simulink model "quadFly"  (R2019b)
settings: Solver=ode4  StartTime=0.0  StopTime=inf  FixedStep=0.001  RelTol=1e-3
InitFcn:
  | Init_control;
values from neighbouring files (symbols this model uses):
  Kd_RP_AgngleRate = 0.005    [Init_control.m]    (also in quadFly.sldd)
  Kd_YAW_AngleRate = 0.05    [Init_control.m]    (also in quadFly.sldd)
  Ki_RP_AgngleRate = 0.01    [Init_control.m]    (also in quadFly.sldd)
  Ki_YAW_AngleRate = 0.8    [Init_control.m]    (also in quadFly.sldd)
  Kp_RP_AgngleRate = 0.55    [Init_control.m]    (also in quadFly.sldd)
  Kp_RP_ANGLE = 6.5    [Init_control.m]    (also in quadFly.sldd)
  Kp_YAW_AngleRate = 3.2    [Init_control.m]    (also in quadFly.sldd)
  MAX_CONTROL_ANGLE_RATE_Y = 90    [Init_control.m]    (also in quadFly.sldd = 90.0)
  ModelInit_RPM = 0.0    [quadFly.sldd]
  ModelParam_envAltitude = -41.5260009765625    [quadFly.sldd]
  ModelParam_GlobalNoiseGainSwitch = 1.0    [quadFly.sldd]
  ModelParam_GPSLatLong = 40.1540302 116.2593683    [quadFly.sldd]
  ModelParam_motorCr = 1148.0    [quadFly.sldd]
  ModelParam_motorJm = 0.0001287    [quadFly.sldd]
  ModelParam_motorMinThr = 0.05    [quadFly.sldd]
  ModelParam_motorT = 0.02    [quadFly.sldd]
  ModelParam_motorWb = -141.4    [quadFly.sldd]
  ModelParam_rotorCm = 1.779E-7    [quadFly.sldd]
  ModelParam_rotorCt = 1.105E-5    [quadFly.sldd]
  ModelParam_uavCCm = 0.01 0.01 0.0055    [quadFly.sldd]
  ModelParam_uavCd = 0.073    [quadFly.sldd]
  ModelParam_uavDearo = 0.12    [quadFly.sldd]
  ModelParam_uavJ = 0.0211 0.0 0.0 0.0 0.0219 0.0 0.0 0.0 0.0366    [quadFly.sldd]
  ModelParam_uavMass = 1.4    [quadFly.sldd]
  ModelParam_uavR = 0.225    [quadFly.sldd]
  ModelParam_uavType = 3    [quadFly.sldd]
undefined symbols (not defined in the file or in its folder): DWORK0, DWORK1, DWORK10, DWORK11, DWORK12, DWORK13, DWORK14, DWORK15, DWORK2, DWORK3, DWORK4, DWORK5, DWORK6, DWORK7, DWORK8, DWORK9, earthRadius, KiPitchAttitude, KiRollAttitude, Receive, Send
libraries: simulink x15, ctrl_ADRC_angular_rate x4, aerolibfltsims x3, ctrl_ADRC_TD x2, shared6dof x1, aerolibanimutils x1
(part 1 of 4)
settings Model: DataDictionary=quadFly.sldd  SimulationMode=accelerator  Creator=dream  LastModifiedBy=75696
settings DataIOCC: ReturnWorkspaceOutputs=off
settings DebuggingCC: BusObjectLabelMismatch=error  ArithmeticOperatorsInVariantConditions=warning
settings SFSimCC: SimUseLocalCustomCode=off  CustomCodeUndefinedFunction=UseInterfaceOnly
settings RTWCC: RTWUseLocalCustomCode=off
settings CodeAppCC: StateflowObjectComments=on

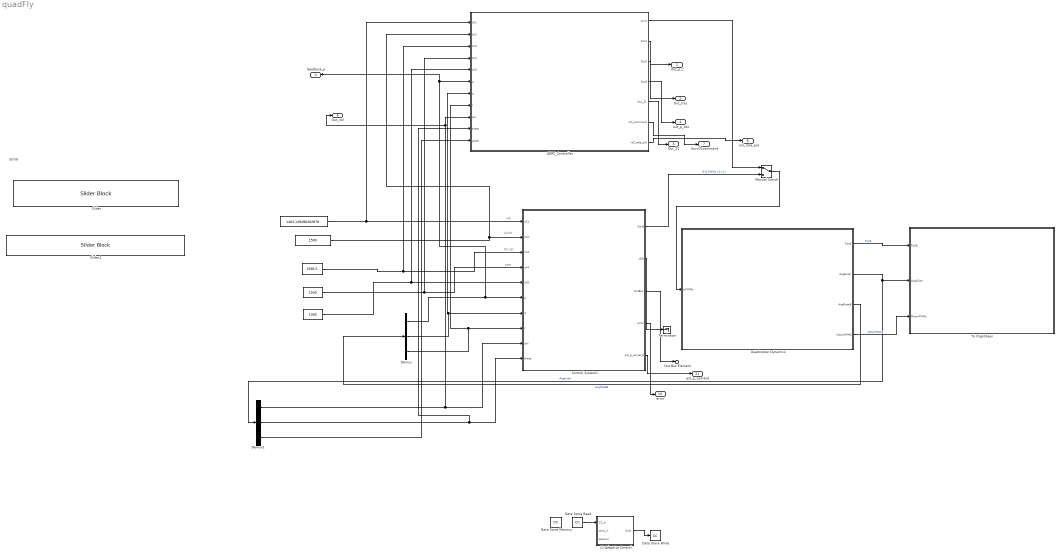
== system quadFly ==
  note: 遥控器
  note: roll
  note: pitch
  note: thrust
  note: yaw
  " " : Constant  Value=1000  OutDataTypeStr=uint16
  "  " : Constant  Value=1500  OutDataTypeStr=uint16
  "   " : Constant  Value=1463.129496402878  OutDataTypeStr=uint16
  "      " : Constant  Value=1596.5  OutDataTypeStr=uint16
  "          " : Constant  Value=1500  OutDataTypeStr=uint16
  "ADRC_Controller " : Subsystem
      mask Display: image('v2-31b439c605ff7f3f51fcae1000b27190_1440w.jpg'); % Use "Edit Image" on toolstrip to change.
  Control System1 : Subsystem
      mask Display: image('icon\pixhawk.png');
  Data Store Memory : DataStoreMemory  DataStoreName=CC  ReadBeforeWriteMsg=warning  WriteAfterWriteMsg=warning  WriteAfterReadMsg=warning  InitialValue=c2init  ShowAdditionalParam=off
  Data Store Read : DataStoreRead  DataStoreName=CC
  Data Store Write : DataStoreWrite  DataStoreName=CC
  Demux : Demux  Outputs=3
  Demux1 : Demux  Outputs=3
  L1-Adaptive Control : Subsystem
  Manual Switch : ManualSwitch
  Quadcopter Dynamics : Subsystem
      mask Display: image('icon/F450.png');
  Slider : SliderBlock  ScaleMin=1100  ScaleMax=1900
  Slider2 : SliderBlock  ScaleMin=1100  ScaleMax=1900
  Terminator : Terminator
  To FlightGear : Subsystem
      mask Display: image('icon/FlightGear.png');
  Out_p_c : Outport
  Out_trac : Outport  Port=2
  feedback_p : Outport  Port=3
  out_p_dot : Outport  Port=4
  Out_Z1 : Outport  Port=5
  Out_roll : Outport  Port=6
  Ouroll1command : Outport  Port=7
  roll_rate_pid : Outport  Port=8
  Out Bus Element : Outport  Port=9  PortName=OutBus  Element=signal1
  error : Outport  Port=10
  pid_p_comand : Outport  Port=11
  wires:
  Quadcopter Dynamics/1(PosE) -> To FlightGear/1(PosE)  "PosE"
  Control System1/2(LED) -> Terminator/1
  Quadcopter Dynamics/2(AngEuler) -> To FlightGear/2(AngEular), Demux1/1  "AngEular"
  "   "/1 -> Control System1/1(ch1), "ADRC_Controller "/1(ch1)
  "          "/1 -> Control System1/4(ch4), "ADRC_Controller "/4(ch4)
  "      "/1 -> "ADRC_Controller "/3(ch3), Control System1/3(ch3)
  Quadcopter Dynamics/3(AngRateB) -> Demux/1  "AngRateB"
  " "/1 -> "ADRC_Controller "/5(ch5), Control System1/5(ch5)
  Demux/1 -> feedback_p/1, "ADRC_Controller "/6(p), Control System1/6(p)
  Demux/2 -> Control System1/7(q), "ADRC_Controller "/7(q)
  Demux/3 -> Control System1/8(r), "ADRC_Controller "/8(r)
  Demux1/1 -> Control System1/9(phi), "ADRC_Controller "/9(phi), Out_roll/1
  Demux1/2 -> "ADRC_Controller "/10(theta), Control System1/10(theta)
  Demux1/3 -> "ADRC_Controller "/11(posai)
  "  "/1 -> "ADRC_Controller "/2(ch2), Control System1/2(ch2)
  Control System1/1(PWM) -> Manual Switch/2  "8-D PWMs（0~1）"
  Quadcopter Dynamics/4(MotorRPMS) -> To FlightGear/3(MotorPWMs)  "MotorPWMs"
  "ADRC_Controller "/1(pwm) -> Manual Switch/1
  Manual Switch/1 -> Quadcopter Dynamics/1(inPWMs)
  "ADRC_Controller "/3(Out2) -> Out_trac/1
  "ADRC_Controller "/2(Out1) -> Out_p_c/1
  "ADRC_Controller "/4(Out3) -> out_p_dot/1
  "ADRC_Controller "/5(Out_Z1) -> Out_Z1/1
  "ADRC_Controller "/6(roll_command) -> Ouroll1command/1
  "ADRC_Controller "/7(roll_rate_pid) -> roll_rate_pid/1
  Control System1/3(OutBus) -> Out Bus Element/1
  Control System1/4(error) -> error/1
  Control System1/5(pid_p_comand) -> pid_p_comand/1
  L1-Adaptive Control/1(Out1) -> Data Store Write/1
  Data Store Read/1 -> L1-Adaptive Control/1(C2_in)

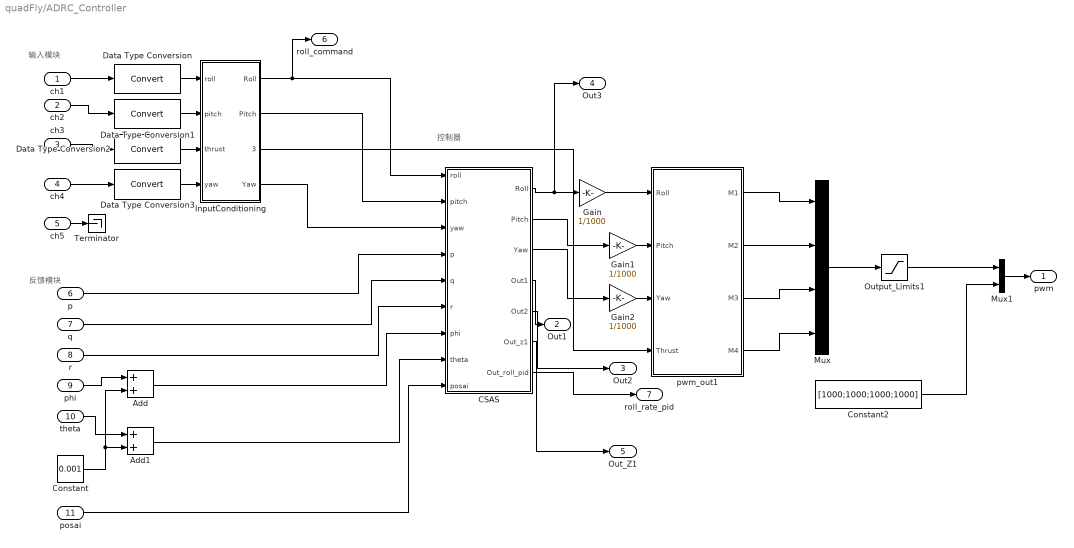
== system quadFly/ADRC_Controller  ==
  note: 控制器
  note: 反馈模块
  note: 输入模块
  ch1 : Inport
  ch2 : Inport  Port=2
  ch3 : Inport  Port=3
  ch4 : Inport  Port=4
  ch5 : Inport  Port=5
  p : Inport  Port=6
  q : Inport  Port=7
  r : Inport  Port=8
  phi : Inport  Port=9
  theta : Inport  Port=10
  posai : Inport  Port=11
  Add : Sum
  Add1 : Sum
  CSAS : Subsystem
  Constant : Constant  Value=0.001
  Constant2 : Constant  Value=[1000;1000;1000;1000]
  Data Type Conversion{,1..3} (4 alike) : DataTypeConversion
  Gain : Gain  Gain=1/1000
  Gain1 : Gain  Gain=1/1000
  Gain2 : Gain  Gain=1/1000
  InputConditioning : Subsystem
  Mux : Mux
  Mux1 : Mux  Inputs=2
  Output_Limits1 : Saturate  UpperLimit=2000  LowerLimit=1000
  Terminator : Terminator
  pwm_out1 : MATLAB Function  TreatAsAtomicUnit=on  SystemSampleTime=0.004
  pwm : Outport
  Out1 : Outport  Port=2
  Out2 : Outport  Port=3
  Out3 : Outport  Port=4
  Out_Z1 : Outport  Port=5
  roll_command : Outport  Port=6
  roll_rate_pid : Outport  Port=7
  wires:
  ch1/1 -> Data Type Conversion/1
  ch2/1 -> Data Type Conversion1/1
  ch3/1 -> Data Type Conversion2/1
  ch4/1 -> Data Type Conversion3/1
  ch5/1 -> Terminator/1
  CSAS/2(Pitch) -> Gain1/1
  Data Type Conversion/1 -> InputConditioning/1(roll)
  Data Type Conversion1/1 -> InputConditioning/2(pitch)
  Data Type Conversion2/1 -> InputConditioning/3(thrust)
  Data Type Conversion3/1 -> InputConditioning/4(yaw)
  phi/1 -> Add/1
  Constant/1 -> Add1/2, Add/2
  theta/1 -> Add1/1
  p/1 -> CSAS/4(p)
  q/1 -> CSAS/5(q)
  r/1 -> CSAS/6(r)
  InputConditioning/1(Roll) -> roll_command/1, CSAS/1(roll)
  InputConditioning/2(Pitch) -> CSAS/2(pitch)
  InputConditioning/4(Yaw) -> CSAS/3(yaw)
  InputConditioning/3(Thrust) -> pwm_out1/4(Thrust)
  Add/1 -> CSAS/7(phi)
  Add1/1 -> CSAS/8(theta)
  CSAS/1(Roll) -> Out3/1, Gain/1
  CSAS/3(Yaw) -> Gain2/1
  Gain/1 -> pwm_out1/1(Roll)
  Gain1/1 -> pwm_out1/2(Pitch)
  Gain2/1 -> pwm_out1/3(Yaw)
  posai/1 -> CSAS/9(posai)
  pwm_out1/2(M2) -> Mux/2
  pwm_out1/1(M1) -> Mux/1
  pwm_out1/3(M3) -> Mux/3
  pwm_out1/4(M4) -> Mux/4
  Mux/1 -> Output_Limits1/1
  Output_Limits1/1 -> Mux1/1
  Constant2/1 -> Mux1/2
  Mux1/1 -> pwm/1
  CSAS/4(Out1) -> Out1/1
  CSAS/5(Out2) -> Out2/1
  CSAS/6(Out_z1) -> Out_Z1/1
  CSAS/7(Out_roll_pid) -> roll_rate_pid/1

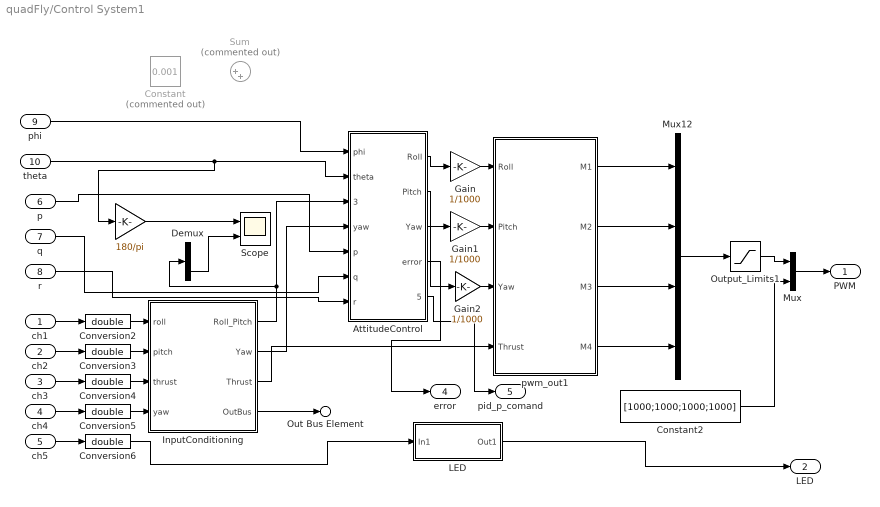
== system quadFly/Control System1 ==
  ch1 : Inport  OutDataTypeStr=uint16  PortDimensions=1
  ch2 : Inport  Port=2  OutDataTypeStr=uint16  PortDimensions=1
  ch3 : Inport  Port=3  OutDataTypeStr=uint16  PortDimensions=1
  ch4 : Inport  Port=4  OutDataTypeStr=uint16  PortDimensions=1
  ch5 : Inport  Port=5  OutDataTypeStr=uint16  PortDimensions=1  Interpolate=off
  p : Inport  Port=6  PortDimensions=1
  q : Inport  Port=7  PortDimensions=1
  r : Inport  Port=8  PortDimensions=1
  phi : Inport  Port=9  PortDimensions=1
  theta : Inport  Port=10  PortDimensions=1
  " " : Gain  Gain=180/pi
  AttitudeControl : Subsystem
  Constant : Constant  Commented=on  Value=0.001
  Constant2 : Constant  Value=[1000;1000;1000;1000]
  Conversion{2..6} (5 alike) : DataTypeConversion  OutDataTypeStr=double
  Demux : Demux  Outputs=2
  Gain : Gain  Gain=1/1000
  Gain1 : Gain  Gain=1/1000
  Gain2 : Gain  Gain=1/1000
  InputConditioning : Subsystem
  "LED " : Subsystem
  Mux : Mux  Inputs=2
  Mux12 : Mux
  Output_Limits1 : Saturate  UpperLimit=2000  LowerLimit=1000
  Scope : Scope  NumInputPorts=2
  Sum : Sum  Commented=on  Inputs=|++
  pwm_out1 : MATLAB Function  TreatAsAtomicUnit=on  SystemSampleTime=0.004
  PWM : Outport  PortDimensions=8  VectorParamsAs1DForOutWhenUnconnected=off
  LED : Outport  Port=2  PortDimensions=1  VectorParamsAs1DForOutWhenUnconnected=off
  Out Bus Element : Outport  Port=3  PortName=OutBus  Element=signal1
  error : Outport  Port=4
  pid_p_comand : Outport  Port=5
  wires:
  InputConditioning/3(Thrust) -> pwm_out1/4(Thrust)
  Mux12/1 -> Output_Limits1/1
  Gain1/1 -> pwm_out1/2(Pitch)
  Gain/1 -> pwm_out1/1(Roll)
  ch3/1 -> Conversion4/1
  pwm_out1/1(M1) -> Mux12/1
  ch5/1 -> Conversion6/1
  pwm_out1/3(M3) -> Mux12/3
  pwm_out1/2(M2) -> Mux12/2
  r/1 -> AttitudeControl/7(r)
  AttitudeControl/1(Roll) -> Gain/1
  Gain2/1 -> pwm_out1/3(Yaw)
  InputConditioning/1(Roll_Pitch) -> Demux/1, AttitudeControl/3(roll_pitch)
  q/1 -> AttitudeControl/6(q)
  InputConditioning/2(Yaw) -> AttitudeControl/4(yaw)
  p/1 -> AttitudeControl/5(p)
  ch4/1 -> Conversion5/1
  pwm_out1/4(M4) -> Mux12/4
  AttitudeControl/3(Yaw) -> Gain2/1
  AttitudeControl/2(Pitch) -> Gain1/1
  ch1/1 -> Conversion2/1
  "LED "/1(Out1) -> LED/1
  ch2/1 -> Conversion3/1
  Conversion6/1 -> "LED "/1(In1)
  Conversion2/1 -> InputConditioning/1(roll)
  Conversion5/1 -> InputConditioning/4(yaw)
  Conversion4/1 -> InputConditioning/3(thrust)
  Conversion3/1 -> InputConditioning/2(pitch)
  " "/1 -> Scope/1
  Demux/2 -> Scope/2
  phi/1 -> AttitudeControl/1(phi)
  theta/1 -> " "/1, AttitudeControl/2(theta)
  Constant2/1 -> Mux/2
  Output_Limits1/1 -> Mux/1
  Mux/1 -> PWM/1
  InputConditioning/4(OutBus) -> Out Bus Element/1
  AttitudeControl/4(error) -> error/1
  AttitudeControl/5(pid_p_comand) -> pid_p_comand/1

== system quadFly/L1-Adaptive Control ==
  C2_in : Inport
  sens_in : Inport  Port=2
  params : Inport  Port=3
  Out1 : Outport
  wires:
  C2_in/1 -> ?

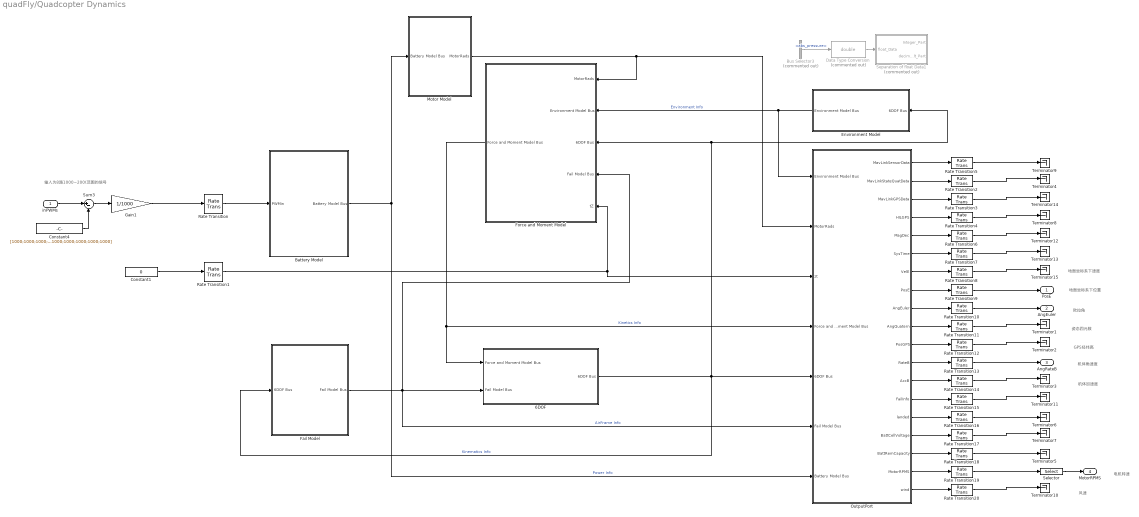
== system quadFly/Quadcopter Dynamics ==
  note: 电机转速
  note: 风速
  note: 机体加速度
  note: 机体角速度
  note: GPS经纬高
  note: 姿态四元数
  note: 欧拉角
  note: 地面坐标系下位置
  note: 地面坐标系下速度
  note: 输入为8路1000~2000范围的信号
  inPWMs : Inport  PortDimensions=8
  6DOF : Subsystem
  Battery Model : Subsystem
      mask help: Simulink:masks:GenSFuncDesc_MD
      mask Help: eval('feval(''rtwprivate'',''rtwhelpview'',''rtw_sfcn_block'')');
  Bus Selector3 : BusSelector  Commented=on  OutputSignals=abs_pressure
  Constant1 : Constant  Value=0
  Constant4 : Constant  Value=[1000;1000;1000;1000;1000;1000;1000;1000]
  Data Type Conversion : DataTypeConversion  Commented=on  OutDataTypeStr=double
  Environment Model : Subsystem  mask{sfcnParam1=ModelParam_GPSLatLong, sfcnParam2=ModelParam_GlobalNoiseGainSwitch, sfcnParam3=ModelParam_envAltitude}
      mask prompts: sfcnParam1 "ModelParam_GPSLatLong:"; sfcnParam2 "ModelParam_GlobalNoiseGainSwitch:"; sfcnParam3 "ModelParam_envAltitude:"
      mask help: Simulink:masks:GenSFuncDesc_MD
      mask Help: eval('feval(''rtwprivate'',''rtwhelpview'',''rtw_sfcn_block'')');
  Fail Model : Subsystem  mask{sfcnParam1=ModelParam_uavJ, sfcnParam2=ModelParam_uavMass, sfcnParam3=ModelParam_uavR}
      mask prompts: sfcnParam1 "ModelParam_uavJ:"; sfcnParam2 "ModelParam_uavMass:"; sfcnParam3 "ModelParam_uavR:"
      mask help: Simulink:masks:GenSFuncDesc_MD
      mask Help: eval('feval(''rtwprivate'',''rtwhelpview'',''rtw_sfcn_block'')');
  Force and Moment Model : Subsystem  mask{sfcnParam1=ModelParam_motorJm, sfcnParam2=ModelParam_rotorCm, sfcnParam3=ModelParam_rotorCt, sfcnParam4=ModelParam_uavCCm, sfcnParam5=ModelParam_uavCd, sfcnParam6=ModelParam_uavDearo, sfcnParam7=ModelParam_uavR, sfcnParam8=ModelParam_uavType}
      mask prompts: sfcnParam1 "ModelParam_motorJm:"; sfcnParam2 "ModelParam_rotorCm:"; sfcnParam3 "ModelParam_rotorCt:"; sfcnParam4 "ModelParam_uavCCm:"; sfcnParam5 "ModelParam_uavCd:"; sfcnParam6 "ModelParam_uavDearo:"; sfcnParam7 "ModelParam_uavR:"; sfcnParam8 "ModelParam_uavType:"
      mask help: Simulink:masks:GenSFuncDesc_MD
      mask Help: eval('feval(''rtwprivate'',''rtwhelpview'',''rtw_sfcn_block'')');
  Gain1 : Gain  Gain=1/1000
  Motor Model : Subsystem  mask{sfcnParam1=ModelInit_RPM, sfcnParam2=ModelParam_motorCr, sfcnParam3=ModelParam_motorMinThr, sfcnParam4=ModelParam_motorT, sfcnParam5=ModelParam_motorWb}
      mask prompts: sfcnParam1 "ModelInit_RPM:"; sfcnParam2 "ModelParam_motorCr:"; sfcnParam3 "ModelParam_motorMinThr:"; sfcnParam4 "ModelParam_motorT:"; sfcnParam5 "ModelParam_motorWb:"
      mask help: Simulink:masks:GenSFuncDesc_MD
      mask Help: eval('feval(''rtwprivate'',''rtwhelpview'',''rtw_sfcn_block'')');
  OutputPort : Subsystem  mask{sfcnParam1=ModelParam_GPSLatLong, sfcnParam2=ModelParam_GlobalNoiseGainSwitch, sfcnParam3=ModelParam_envAltitude}
      mask prompts: sfcnParam1 "ModelParam_GPSLatLong:"; sfcnParam2 "ModelParam_GlobalNoiseGainSwitch:"; sfcnParam3 "ModelParam_envAltitude:"
      mask help: Simulink:masks:GenSFuncDesc_MD
      mask Help: eval('feval(''rtwprivate'',''rtwhelpview'',''rtw_sfcn_block'')');
  Rate Transition{,1..20} (21 alike) : RateTransition  OutPortSampleTime=ModelParam_BusSampleRate
  Selector : Selector  InputPortWidth=8  IndexOptions=Index vector (dialog)  Indices=[1 2 3 4]  OutputSizes=1
  Separation of float Data1 : Subsystem  Commented=on  mask{IntUint=1}
      mask prompts: IntUint "整数单位"
      mask help: 分离浮点数的整数和小数部分，这样在Labview MIT模块中可以稳定输出精度
  Sum3 : Sum  Inputs=|+-
  Terminator{1..15} (15 alike) : Terminator
  PosE : Outport  VectorParamsAs1DForOutWhenUnconnected=off
  AngEuler : Outport  Port=2  VectorParamsAs1DForOutWhenUnconnected=off
  AngRateB : Outport  Port=3  VectorParamsAs1DForOutWhenUnconnected=off
  MotorRPMS : Outport  Port=4  VectorParamsAs1DForOutWhenUnconnected=off
  wires:
  Selector/1 -> MotorRPMS/1
  Constant4/1 -> Sum3/2
  inPWMs/1 -> Sum3/1
  Constant1/1 -> Rate Transition1/1
  Sum3/1 -> Gain1/1
  Rate Transition5/1 -> Terminator9/1
  Rate Transition2/1 -> Terminator4/1
  Rate Transition3/1 -> Terminator14/1
  Rate Transition4/1 -> Terminator8/1
  Rate Transition6/1 -> Terminator12/1
  Rate Transition7/1 -> Terminator13/1
  Rate Transition8/1 -> Terminator15/1
  Rate Transition9/1 -> PosE/1
  Rate Transition10/1 -> AngEuler/1
  Rate Transition11/1 -> Terminator1/1
  Rate Transition12/1 -> Terminator2/1
  Rate Transition13/1 -> AngRateB/1
  Rate Transition14/1 -> Terminator3/1
  Rate Transition15/1 -> Terminator11/1
  Rate Transition16/1 -> Terminator6/1
  Rate Transition17/1 -> Terminator7/1
  Rate Transition18/1 -> Terminator5/1
  Rate Transition19/1 -> Selector/1
  Rate Transition20/1 -> Terminator10/1
  Gain1/1 -> Rate Transition/1
  OutputPort/2(MavLinkStateQuatData) -> Rate Transition2/1
  Motor Model/1(MotorRads) -> OutputPort/2(MotorRads), Force and Moment Model/1(MotorRads)
  OutputPort/15(landed) -> Rate Transition16/1
  OutputPort/3(MavLinkGPSData) -> Rate Transition3/1
  Bus Selector3/1 -> Data Type Conversion/1  "<abs_pressure>"
  Data Type Conversion/1 -> Separation of float Data1/1(float_Data)
  OutputPort/1(MavLinkSensorData) -> Rate Transition5/1
  OutputPort/14(FailInfo) -> Rate Transition15/1
  OutputPort/13(AccB) -> Rate Transition14/1
  OutputPort/12(RateB) -> Rate Transition13/1
  OutputPort/11(PosGPS) -> Rate Transition12/1
  OutputPort/10(AngQuatern) -> Rate Transition11/1
  OutputPort/9(AngEuler) -> Rate Transition10/1
  OutputPort/8(PosE) -> Rate Transition9/1
  OutputPort/7(VelE) -> Rate Transition8/1
  OutputPort/6(SysTime) -> Rate Transition7/1
  OutputPort/5(MagDec) -> Rate Transition6/1
  OutputPort/4(HILGPS) -> Rate Transition4/1
  Battery Model/1(Battery Model Bus) -> OutputPort/7(Battery Model Bus), Motor Model/1(Battery Model Bus)  "Power Info"
  Fail Model/1(Fail Model Bus) -> OutputPort/6(Fail Model Bus), Force and Moment Model/4(Fail Model Bus), 6DOF/2(Fail Model Bus)  "AirFrame Info"
  Force and Moment Model/1(Force and Moment Model Bus) -> OutputPort/4(Force and Moment Model Bus), 6DOF/1(Force and Moment Model Bus)  "Kinetics Info"
  6DOF/1(6DOF Bus) -> OutputPort/5(6DOF Bus), Fail Model/1(6DOF Bus), Environment Model/1(6DOF Bus), Force and Moment Model/3(6DOF Bus)  "Kinematics Info"
  Environment Model/1(Environment Model Bus) -> OutputPort/1(Environment Model Bus), Force and Moment Model/2(Environment Model Bus)  "Environment Info"
  OutputPort/16(BattCellVoltage) -> Rate Transition17/1
  OutputPort/17(BattRemCapacity) -> Rate Transition18/1
  OutputPort/19(wind) -> Rate Transition20/1
  OutputPort/18(MotorRPMS) -> Rate Transition19/1
  Rate Transition/1 -> Battery Model/1(PWMin)
  Rate Transition1/1 -> OutputPort/3(zt), Force and Moment Model/5("tZ ")

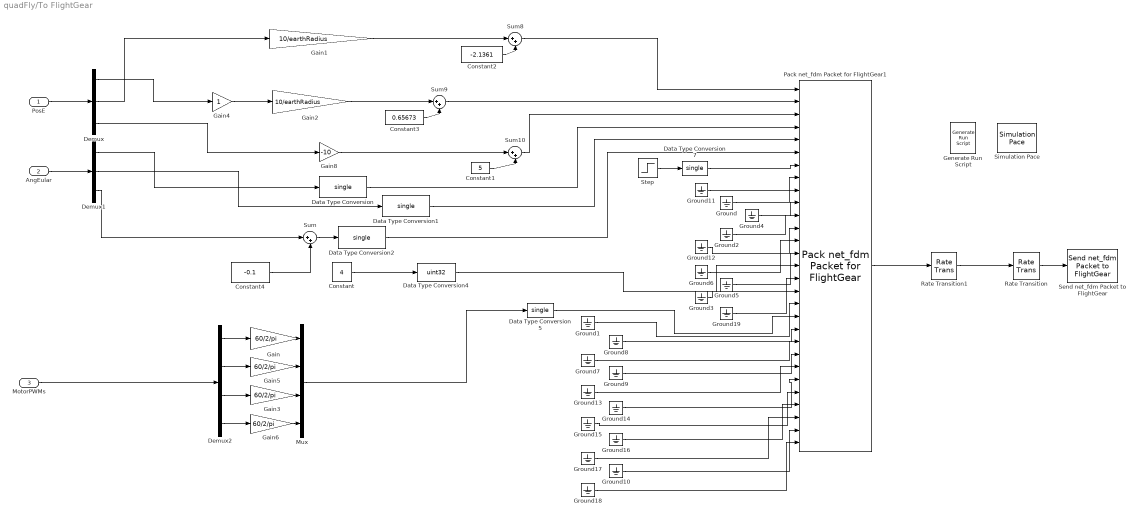
== system quadFly/To FlightGear ==
  PosE : Inport
  AngEular : Inport  Port=2
  MotorPWMs : Inport  Port=3
  Constant : Constant  Value=4
  Constant1 : Constant  Value=5  VectorParams1D=off
  Constant2 : Constant  Value=-2.1361  VectorParams1D=off
  Constant3 : Constant  Value=0.65673  VectorParams1D=off
  Constant4 : Constant  Value=-0.1  VectorParams1D=off
  Data Type Conversion : DataTypeConversion  OutDataTypeStr=single  SaturateOnIntegerOverflow=on
  Data Type Conversion1 : DataTypeConversion  OutDataTypeStr=single  SaturateOnIntegerOverflow=on
  Data Type Conversion2 : DataTypeConversion  OutDataTypeStr=single  SaturateOnIntegerOverflow=on
  Data Type Conversion4 : DataTypeConversion  OutDataTypeStr=uint32
  Data Type Conversion5 : DataTypeConversion  OutDataTypeStr=single
  Data Type Conversion7 : DataTypeConversion  OutDataTypeStr=single
  Demux : Demux  Outputs=3
  Demux1 : Demux  Outputs=3
  Demux2 : Demux
  Gain{,3,5..6} (4 alike) : Gain  Gain=60/2/pi
  Gain1 : Gain  Gain=10/earthRadius
  Gain2 : Gain  Gain=10/earthRadius
  Gain4 : Gain
  Gain8 : Gain  Gain=-10
  Generate Run Script : aerolibfltsims/Generate Run Script  Architecture=Default  dataFlow=Send-Receive  GeometryModelName=Rotor4  AirportId=KSF0  RunwayId=10L  InitialAltitude=0  InitialHeading=0  OffsetDistance=0  OffsetAzimuth=0  InstallScenery=off  DisableShaders=off  OriginAddress=127.0.0.1  DestinationPort=5502  OriginPort=5505  LocalAddress=127.0.0.1  OutputFileName=runfg.bat  FlightGearBaseDirectory=C:\Program Files\FlightGear 2016.1.2
  Ground{,1..19} (20 alike) : Ground
  Mux : Mux
  Pack net_fdm Packet for FlightGear1 : aerolibfltsims/Pack net_fdm Packet for FlightGear  FlightGearVersion=v2016.1  ShowPositionAttitudeInputs=on  ShowVelocityAccelerationInputs=off  ShowControlSurfacePositionInputs=on  ShowEngineFuelInputs=on  ShowLandingGearInputs=off  ShowEnvironmentInputs=off  SampleTime=0.01  packetVersion=24
      settings: SourceProductName=Aerospace Blockset  SourceProductBaseCode=AE
  Rate Transition : RateTransition
  Rate Transition1 : RateTransition
  Send net_fdm Packet to FlightGear : aerolibfltsims/Send net_fdm Packet to FlightGear  DestinationIpAddress=127.0.0.1  DestinationPort=5502  LocalIpPort=-1  varLen=off  SampleTime=0.005
      settings: SourceProductName=Aerospace Blockset  SourceProductBaseCode=AE
  Simulation Pace : aerolibanimutils/Simulation Pace  SimulationPace=1  SleepMode=MATLAB Thread  OutputPaceError=off  SampleTime=-1
      settings: AttributesFormatString=%<SimulationPace> sec/sec
  Step : Step  Time=5  SampleTime=0
  Sum{,8..10} (4 alike) : Sum  Inputs=|++
  wires:
  Rate Transition/1 -> Send net_fdm Packet to FlightGear/1
  Demux/1 -> Gain4/1
  Demux/2 -> Gain1/1
  Demux/3 -> Gain8/1
  Constant4/1 -> Sum/2
  Sum/1 -> Data Type Conversion2/1
  Gain1/1 -> Sum8/1
  Constant2/1 -> Sum8/2
  Gain2/1 -> Sum9/1
  Constant3/1 -> Sum9/2
  Constant1/1 -> Sum10/2
  Gain8/1 -> Sum10/1
  Pack net_fdm Packet for FlightGear1/1 -> Rate Transition1/1
  Demux1/2 -> Data Type Conversion1/1
  Demux1/3 -> Sum/1
  Data Type Conversion7/1 -> Pack net_fdm Packet for FlightGear1/7
  Ground8/1 -> Pack net_fdm Packet for FlightGear1/20
  Ground/1 -> Pack net_fdm Packet for FlightGear1/9
  Ground7/1 -> Pack net_fdm Packet for FlightGear1/21
  Ground9/1 -> Pack net_fdm Packet for FlightGear1/22
  Ground13/1 -> Pack net_fdm Packet for FlightGear1/23
  Ground14/1 -> Pack net_fdm Packet for FlightGear1/24
  Ground15/1 -> Pack net_fdm Packet for FlightGear1/25
  Ground16/1 -> Pack net_fdm Packet for FlightGear1/26
  Ground17/1 -> Pack net_fdm Packet for FlightGear1/27
  Ground10/1 -> Pack net_fdm Packet for FlightGear1/28
  Ground18/1 -> Pack net_fdm Packet for FlightGear1/29
  Step/1 -> Data Type Conversion7/1
  Data Type Conversion4/1 -> Pack net_fdm Packet for FlightGear1/17
  Ground1/1 -> Pack net_fdm Packet for FlightGear1/18
  Ground3/1 -> Pack net_fdm Packet for FlightGear1/15
  Ground5/1 -> Pack net_fdm Packet for FlightGear1/14
  Ground6/1 -> Pack net_fdm Packet for FlightGear1/13
  Ground4/1 -> Pack net_fdm Packet for FlightGear1/10
  Ground11/1 -> Pack net_fdm Packet for FlightGear1/8
  Data Type Conversion2/1 -> Pack net_fdm Packet for FlightGear1/6
  Data Type Conversion1/1 -> Pack net_fdm Packet for FlightGear1/5
  Data Type Conversion/1 -> Pack net_fdm Packet for FlightGear1/4
  Sum8/1 -> Pack net_fdm Packet for FlightGear1/1
  Sum9/1 -> Pack net_fdm Packet for FlightGear1/2
  Sum10/1 -> Pack net_fdm Packet for FlightGear1/3
  Constant/1 -> Data Type Conversion4/1
  Data Type Conversion5/1 -> Pack net_fdm Packet for FlightGear1/19
  Ground2/1 -> Pack net_fdm Packet for FlightGear1/11
  Ground12/1 -> Pack net_fdm Packet for FlightGear1/12
  Ground19/1 -> Pack net_fdm Packet for FlightGear1/16
  Gain4/1 -> Gain2/1
  AngEular/1 -> Demux1/1
  PosE/1 -> Demux/1
  MotorPWMs/1 -> Demux2/1
  Mux/1 -> Data Type Conversion5/1
  Demux2/1 -> Gain/1
  Demux2/3 -> Gain3/1
  Gain/1 -> Mux/1
  Gain3/1 -> Mux/3
  Demux2/2 -> Gain5/1
  Gain5/1 -> Mux/2
  Demux2/4 -> Gain6/1
  Gain6/1 -> Mux/4
  Demux1/1 -> Data Type Conversion/1
  Rate Transition1/1 -> Rate Transition/1

== system quadFly/ADRC_Controller /CSAS ==
  note: 角速度反馈
  note: 角速度环_ADRC
  note: 角度环_PID
  note: 角度反馈
  note: 角度指令
  roll : Inport
  pitch : Inport  Port=2
  yaw : Inport  Port=3
  p : Inport  Port=4
  q : Inport  Port=5
  r : Inport  Port=6
  phi : Inport  Port=7
  theta : Inport  Port=8
  posai : Inport  Port=9
  Ground : Ground
  Ground1 : Ground
  Terminator : Terminator
  Terminator1 : Terminator
  angularRate_ADRC : Subsystem
  angular_PID : Subsystem
  Roll : Outport
  Pitch : Outport  Port=2
  Yaw : Outport  Port=3
  Out1 : Outport  Port=4
  Out2 : Outport  Port=5
  Out_z1 : Outport  Port=6
  Out_roll_pid : Outport  Port=7
  wires:
  roll/1 -> angular_PID/1(Roll)
  pitch/1 -> angular_PID/2(Pitch)
  yaw/1 -> angularRate_ADRC/4(yawrate)
  p/1 -> angularRate_ADRC/2(p)
  angularRate_ADRC/1(Roll_U) -> Roll/1
  angularRate_ADRC/2(Pitch_U) -> Pitch/1
  angularRate_ADRC/3(Yaw_U) -> Yaw/1
  phi/1 -> angular_PID/3(phi)
  theta/1 -> angular_PID/4(theta)
  posai/1 -> Terminator/1
  angular_PID/1(roll_rate) -> angularRate_ADRC/1(rollrate), Out_roll_pid/1
  r/1 -> angularRate_ADRC/6(R)
  q/1 -> angularRate_ADRC/5(q)
  angular_PID/2(pitch_rate) -> angularRate_ADRC/3(pitchrate)
  angular_PID/3(yaw_rate) -> Terminator1/1
  Ground/1 -> angular_PID/5(posai)
  Ground1/1 -> angular_PID/6(yaw)
  angularRate_ADRC/4(Out1) -> Out1/1
  angularRate_ADRC/5(Out2) -> Out2/1
  angularRate_ADRC/6(Out_z1) -> Out_z1/1

== system quadFly/ADRC_Controller /InputConditioning ==
  roll : Inport
  pitch : Inport  Port=2
  thrust : Inport  Port=3
  yaw : Inport  Port=4
  Fcn2 : Fcn  Expr=(u - 1500) / 800
  Fcn5 : Fcn  Expr=(u - 1500) / 800
  Fcn6 : Fcn  Expr=(u - 1100) / 800
  Fcn7 : Fcn  Expr=(u - 1500) / 800
  Gain : Gain  Gain=MAX_CONTROL_ANGLE_RATE_Y
  Gain1 : Gain  Gain=3.1415
  Gain2 : Gain  Gain=3.1415
  MATLAB Function : MATLAB Function  TreatAsAtomicUnit=on
  MATLAB Function1 : MATLAB Function  TreatAsAtomicUnit=on
  MATLAB Function2 : MATLAB Function  TreatAsAtomicUnit=on
  MATLAB Function3 : MATLAB Function  TreatAsAtomicUnit=on
  Saturation10 : Saturate  UpperLimit=1  LowerLimit=0
  Saturation7 : Saturate  UpperLimit=1  LowerLimit=-1
  Saturation8 : Saturate  UpperLimit=1  LowerLimit=-1
  Saturation9 : Saturate  UpperLimit=1  LowerLimit=-1
  Roll : Outport  VectorParamsAs1DForOutWhenUnconnected=off
  Pitch : Outport  Port=2  VectorParamsAs1DForOutWhenUnconnected=off
  Thrust : Outport  Port=3  VectorParamsAs1DForOutWhenUnconnected=off
  Yaw : Outport  Port=4  VectorParamsAs1DForOutWhenUnconnected=off
  wires:
  Saturation10/1 -> Thrust/1
  Saturation7/1 -> Gain/1
  Saturation8/1 -> Gain2/1
  Fcn6/1 -> Saturation10/1
  Fcn2/1 -> Saturation9/1
  Fcn5/1 -> Saturation8/1
  Saturation9/1 -> Gain1/1
  Fcn7/1 -> Saturation7/1
  pitch/1 -> MATLAB Function2/1(u)
  MATLAB Function1/1(y) -> Fcn7/1
  thrust/1 -> MATLAB Function3/1(u)
  roll/1 -> MATLAB Function/1(u)
  MATLAB Function2/1(y) -> Fcn5/1
  MATLAB Function/1(y) -> Fcn2/1
  yaw/1 -> MATLAB Function1/1(u)
  MATLAB Function3/1(y) -> Fcn6/1
  Gain/1 -> Yaw/1
  Gain1/1 -> Roll/1
  Gain2/1 -> Pitch/1

== system quadFly/Control System1/AttitudeControl ==
  phi : Inport
  theta : Inport  Port=2
  roll_pitch : Inport  Port=3
  yaw : Inport  Port=4
  p : Inport  Port=5
  q : Inport  Port=6
  r : Inport  Port=7
  "          " : Gain  Gain=180/pi
  Demux12 : Demux  Outputs=2
  Demux16 : Demux  Outputs=2
  Mux22 : Mux  Inputs=2
  Sum{17..19,21..22} (5 alike) : Sum  Inputs=|-+
  pitch_attitude : simulink/Continuous/PID Controller  Controller=P  Form=Parallel  TimeDomain=Discrete-time  SampleTime=-1  IntegratorMethod=Forward Euler  FilterMethod=Forward Euler  ControllerParametersSource=internal  P=Kp_RP_ANGLE  I=KiPitchAttitude  D=0.01  UseFilter=on  N=100  TunerSelectOption=Transfer Function Based (PID Tuner App)  InitialConditionSource=internal  InitialConditionForIntegrator=0  InitialConditionForFilter=0  DifferentiatorICPrevScaledInput=0  ExternalReset=none  TrackingMode=off  Kt=1  LimitOutput=on  UpperSaturationLimit=180  LowerSaturationLimit=-180  LinearizeAsGain=on  AntiWindupMode=back-calculation  Kb=1  POutMin=[]  POutMax=[]  IOutMin=[]  IOutMax=[]  DOutMin=[]  DOutMax=[]  NOutMin=[]  NOutMax=[]  SumOutMin=[]  SumOutMax=[]  SaturationOutMin=[]  SaturationOutMax=[]  PParamMin=[]  PParamMax=[]  IParamMin=[]  IParamMax=[]  DParamMin=[]  DParamMax=[]  NParamMin=[]  NParamMax=[]  KbParamMin=[]  KbParamMax=[]  KtParamMin=[]  KtParamMax=[]  KbOutMin=[]  KbOutMax=[]  KtOutMin=[]  KtOutMax=[]  IntegratorOutMin=[]  IntegratorOutMax=[]  FilterOutMin=[]  FilterOutMax=[]  SumI1OutMin=[]  SumI1OutMax=[]  SumI2OutMin=[]  SumI2OutMax=[]  SumI3OutMin=[]  SumI3OutMax=[]  SumI4OutMin=[]  SumI4OutMax=[]  SumDOutMin=[]  SumDOutMax=[]  DifferentiatorOutMin=[]  DifferentiatorOutMax=[]  FilterDiffOutCoefMin=[]  FilterDiffOutCoefMax=[]  ReciprocalOutMin=[]  ReciprocalOutMax=[]  SumDenOutMin=[]  SumDenOutMax=[]  SumNumOutMin=[]  SumNumOutMax=[]  DivideOutMin=[]  DivideOutMax=[]  IntegratorContinuousStateAttributes=''  IntegratorStateMustResolveToSignalObject=off  IntegratorRTWStateStorageClass=Auto  FilterContinuousStateAttributes=''  FilterStateMustResolveToSignalObject=off  FilterRTWStateStorageClass=Auto  ParallelPVariant=InternalParameters  IdealPVariant=Disabled  IVariant=Disabled  DVariant=Disabled  IntegratorVariant=Disabled  SatVariant=Enabled  AWVariant=Disabled  PCopyVariant=Disabled  TRVariant=Disabled  FdbkBlocksVariant=Forward  IdealPFdbkVariant=Disabled  SatFdbkVariant=Disabled  DerivativeFilterVariant=Disabled  NVariant=Disabled  NCopyVariant=Disabled_SignalSpec  FilterICVariant=Disabled  IntegratorICVariant=Disabled  ExternalResetVariant=Disabled  TRSumVariant=Passthrough  SumFdbkVariant=Disabled  SumVariant=Passthrough_P
  pitch_rate : simulink/Continuous/PID Controller  Controller=PID  Form=Parallel  TimeDomain=Discrete-time  SampleTime=-1  IntegratorMethod=Forward Euler  FilterMethod=Forward Euler  ControllerParametersSource=internal  P=60  I=Ki_RP_AgngleRate  D=Kd_RP_AgngleRate  UseFilter=off  N=100  TunerSelectOption=Transfer Function Based (PID Tuner App)  InitialConditionSource=internal  InitialConditionForIntegrator=0  InitialConditionForFilter=0  DifferentiatorICPrevScaledInput=0  ExternalReset=none  TrackingMode=off  Kt=1  LimitOutput=on  UpperSaturationLimit=500  LowerSaturationLimit=-500  LinearizeAsGain=on  AntiWindupMode=back-calculation  Kb=1  POutMin=[]  POutMax=[]  IOutMin=[]  IOutMax=[]  DOutMin=[]  DOutMax=[]  NOutMin=[]  NOutMax=[]  SumOutMin=[]  SumOutMax=[]  SaturationOutMin=[]  SaturationOutMax=[]  PParamMin=[]  PParamMax=[]  IParamMin=[]  IParamMax=[]  DParamMin=[]  DParamMax=[]  NParamMin=[]  NParamMax=[]  KbParamMin=[]  KbParamMax=[]  KtParamMin=[]  KtParamMax=[]  KbOutMin=[]  KbOutMax=[]  KtOutMin=[]  KtOutMax=[]  IntegratorOutMin=[]  IntegratorOutMax=[]  FilterOutMin=[]  FilterOutMax=[]  SumI1OutMin=[]  SumI1OutMax=[]  SumI2OutMin=[]  SumI2OutMax=[]  SumI3OutMin=[]  SumI3OutMax=[]  SumI4OutMin=[]  SumI4OutMax=[]  SumDOutMin=[]  SumDOutMax=[]  DifferentiatorOutMin=[]  DifferentiatorOutMax=[]  FilterDiffOutCoefMin=[]  FilterDiffOutCoefMax=[]  ReciprocalOutMin=[]  ReciprocalOutMax=[]  SumDenOutMin=[]  SumDenOutMax=[]  SumNumOutMin=[]  SumNumOutMax=[]  DivideOutMin=[]  DivideOutMax=[]  IntegratorContinuousStateAttributes=''  IntegratorStateMustResolveToSignalObject=off  IntegratorRTWStateStorageClass=Auto  FilterContinuousStateAttributes=''  FilterStateMustResolveToSignalObject=off  FilterRTWStateStorageClass=Auto  ParallelPVariant=InternalParameters  IdealPVariant=Disabled  IVariant=InternalParameters  DVariant=InternalParameters  IntegratorVariant=Discrete  SatVariant=Enabled  AWVariant=BackCalculation  PCopyVariant=Disabled  TRVariant=Disabled  FdbkBlocksVariant=Forward  IdealPFdbkVariant=Disabled  SatFdbkVariant=Disabled  DerivativeFilterVariant=Differentiator  NVariant=Passthrough  NCopyVariant=Disabled_SignalSpec  FilterICVariant=InternalICsDifferentiator  IntegratorICVariant=InternalICs  ExternalResetVariant=Disabled  TRSumVariant=Passthrough  SumFdbkVariant=Disabled  SumVariant=Sum_PID
  roll_attitude : simulink/Continuous/PID Controller  Controller=P  Form=Parallel  TimeDomain=Discrete-time  SampleTime=-1  IntegratorMethod=Forward Euler  FilterMethod=Forward Euler  ControllerParametersSource=internal  P=6.5  I=100  D=0.01  UseFilter=on  N=100  TunerSelectOption=Transfer Function Based (PID Tuner App)  InitialConditionSource=internal  InitialConditionForIntegrator=0  InitialConditionForFilter=0  DifferentiatorICPrevScaledInput=0  ExternalReset=none  TrackingMode=off  Kt=1  LimitOutput=on  UpperSaturationLimit=180  LowerSaturationLimit=-180  LinearizeAsGain=on  AntiWindupMode=back-calculation  Kb=1  POutMin=[]  POutMax=[]  IOutMin=[]  IOutMax=[]  DOutMin=[]  DOutMax=[]  NOutMin=[]  NOutMax=[]  SumOutMin=[]  SumOutMax=[]  SaturationOutMin=[]  SaturationOutMax=[]  PParamMin=[]  PParamMax=[]  IParamMin=[]  IParamMax=[]  DParamMin=[]  DParamMax=[]  NParamMin=[]  NParamMax=[]  KbParamMin=[]  KbParamMax=[]  KtParamMin=[]  KtParamMax=[]  KbOutMin=[]  KbOutMax=[]  KtOutMin=[]  KtOutMax=[]  IntegratorOutMin=[]  IntegratorOutMax=[]  FilterOutMin=[]  FilterOutMax=[]  SumI1OutMin=[]  SumI1OutMax=[]  SumI2OutMin=[]  SumI2OutMax=[]  SumI3OutMin=[]  SumI3OutMax=[]  SumI4OutMin=[]  SumI4OutMax=[]  SumDOutMin=[]  SumDOutMax=[]  DifferentiatorOutMin=[]  DifferentiatorOutMax=[]  FilterDiffOutCoefMin=[]  FilterDiffOutCoefMax=[]  ReciprocalOutMin=[]  ReciprocalOutMax=[]  SumDenOutMin=[]  SumDenOutMax=[]  SumNumOutMin=[]  SumNumOutMax=[]  DivideOutMin=[]  DivideOutMax=[]  IntegratorContinuousStateAttributes=''  IntegratorStateMustResolveToSignalObject=off  IntegratorRTWStateStorageClass=Auto  FilterContinuousStateAttributes=''  FilterStateMustResolveToSignalObject=off  FilterRTWStateStorageClass=Auto  ParallelPVariant=InternalParameters  IdealPVariant=Disabled  IVariant=Disabled  DVariant=Disabled  IntegratorVariant=Disabled  SatVariant=Enabled  AWVariant=Disabled  PCopyVariant=Disabled  TRVariant=Disabled  FdbkBlocksVariant=Forward  IdealPFdbkVariant=Disabled  SatFdbkVariant=Disabled  DerivativeFilterVariant=Disabled  NVariant=Disabled  NCopyVariant=Disabled_SignalSpec  FilterICVariant=Disabled  IntegratorICVariant=Disabled  ExternalResetVariant=Disabled  TRSumVariant=Passthrough  SumFdbkVariant=Disabled  SumVariant=Passthrough_P
  roll_rate : simulink/Continuous/PID Controller  Controller=PID  Form=Parallel  TimeDomain=Discrete-time  SampleTime=-1  IntegratorMethod=Forward Euler  FilterMethod=Forward Euler  ControllerParametersSource=internal  P=60  I=Ki_RP_AgngleRate  D=Kd_RP_AgngleRate  UseFilter=off  N=100  TunerSelectOption=Transfer Function Based (PID Tuner App)  InitialConditionSource=internal  InitialConditionForIntegrator=0  InitialConditionForFilter=0  DifferentiatorICPrevScaledInput=0  ExternalReset=none  TrackingMode=off  Kt=1  LimitOutput=on  UpperSaturationLimit=500  LowerSaturationLimit=-500  LinearizeAsGain=on  AntiWindupMode=back-calculation  Kb=1  POutMin=[]  POutMax=[]  IOutMin=[]  IOutMax=[]  DOutMin=[]  DOutMax=[]  NOutMin=[]  NOutMax=[]  SumOutMin=[]  SumOutMax=[]  SaturationOutMin=[]  SaturationOutMax=[]  PParamMin=[]  PParamMax=[]  IParamMin=[]  IParamMax=[]  DParamMin=[]  DParamMax=[]  NParamMin=[]  NParamMax=[]  KbParamMin=[]  KbParamMax=[]  KtParamMin=[]  KtParamMax=[]  KbOutMin=[]  KbOutMax=[]  KtOutMin=[]  KtOutMax=[]  IntegratorOutMin=[]  IntegratorOutMax=[]  FilterOutMin=[]  FilterOutMax=[]  SumI1OutMin=[]  SumI1OutMax=[]  SumI2OutMin=[]  SumI2OutMax=[]  SumI3OutMin=[]  SumI3OutMax=[]  SumI4OutMin=[]  SumI4OutMax=[]  SumDOutMin=[]  SumDOutMax=[]  DifferentiatorOutMin=[]  DifferentiatorOutMax=[]  FilterDiffOutCoefMin=[]  FilterDiffOutCoefMax=[]  ReciprocalOutMin=[]  ReciprocalOutMax=[]  SumDenOutMin=[]  SumDenOutMax=[]  SumNumOutMin=[]  SumNumOutMax=[]  DivideOutMin=[]  DivideOutMax=[]  IntegratorContinuousStateAttributes=''  IntegratorStateMustResolveToSignalObject=off  IntegratorRTWStateStorageClass=Auto  FilterContinuousStateAttributes=''  FilterStateMustResolveToSignalObject=off  FilterRTWStateStorageClass=Auto  ParallelPVariant=InternalParameters  IdealPVariant=Disabled  IVariant=InternalParameters  DVariant=InternalParameters  IntegratorVariant=Discrete  SatVariant=Enabled  AWVariant=BackCalculation  PCopyVariant=Disabled  TRVariant=Disabled  FdbkBlocksVariant=Forward  IdealPFdbkVariant=Disabled  SatFdbkVariant=Disabled  DerivativeFilterVariant=Differentiator  NVariant=Passthrough  NCopyVariant=Disabled_SignalSpec  FilterICVariant=InternalICsDifferentiator  IntegratorICVariant=InternalICs  ExternalResetVariant=Disabled  TRSumVariant=Passthrough  SumFdbkVariant=Disabled  SumVariant=Sum_PID
  yaw_rate : simulink/Continuous/PID Controller  Controller=PID  Form=Parallel  TimeDomain=Discrete-time  SampleTime=-1  IntegratorMethod=Forward Euler  FilterMethod=Forward Euler  ControllerParametersSource=internal  P=Kp_YAW_AngleRate  I=Ki_YAW_AngleRate  D=Kd_YAW_AngleRate  UseFilter=off  N=100  TunerSelectOption=Transfer Function Based (PID Tuner App)  InitialConditionSource=internal  InitialConditionForIntegrator=0  InitialConditionForFilter=0  DifferentiatorICPrevScaledInput=0  ExternalReset=none  TrackingMode=off  Kt=1  LimitOutput=on  UpperSaturationLimit=500  LowerSaturationLimit=-500  LinearizeAsGain=on  AntiWindupMode=back-calculation  Kb=1  POutMin=[]  POutMax=[]  IOutMin=[]  IOutMax=[]  DOutMin=[]  DOutMax=[]  NOutMin=[]  NOutMax=[]  SumOutMin=[]  SumOutMax=[]  SaturationOutMin=[]  SaturationOutMax=[]  PParamMin=[]  PParamMax=[]  IParamMin=[]  IParamMax=[]  DParamMin=[]  DParamMax=[]  NParamMin=[]  NParamMax=[]  KbParamMin=[]  KbParamMax=[]  KtParamMin=[]  KtParamMax=[]  KbOutMin=[]  KbOutMax=[]  KtOutMin=[]  KtOutMax=[]  IntegratorOutMin=[]  IntegratorOutMax=[]  FilterOutMin=[]  FilterOutMax=[]  SumI1OutMin=[]  SumI1OutMax=[]  SumI2OutMin=[]  SumI2OutMax=[]  SumI3OutMin=[]  SumI3OutMax=[]  SumI4OutMin=[]  SumI4OutMax=[]  SumDOutMin=[]  SumDOutMax=[]  DifferentiatorOutMin=[]  DifferentiatorOutMax=[]  FilterDiffOutCoefMin=[]  FilterDiffOutCoefMax=[]  ReciprocalOutMin=[]  ReciprocalOutMax=[]  SumDenOutMin=[]  SumDenOutMax=[]  SumNumOutMin=[]  SumNumOutMax=[]  DivideOutMin=[]  DivideOutMax=[]  IntegratorContinuousStateAttributes=''  IntegratorStateMustResolveToSignalObject=off  IntegratorRTWStateStorageClass=Auto  FilterContinuousStateAttributes=''  FilterStateMustResolveToSignalObject=off  FilterRTWStateStorageClass=Auto  ParallelPVariant=InternalParameters  IdealPVariant=Disabled  IVariant=InternalParameters  DVariant=InternalParameters  IntegratorVariant=Discrete  SatVariant=Enabled  AWVariant=BackCalculation  PCopyVariant=Disabled  TRVariant=Disabled  FdbkBlocksVariant=Forward  IdealPFdbkVariant=Disabled  SatFdbkVariant=Disabled  DerivativeFilterVariant=Differentiator  NVariant=Passthrough  NCopyVariant=Disabled_SignalSpec  FilterICVariant=InternalICsDifferentiator  IntegratorICVariant=InternalICs  ExternalResetVariant=Disabled  TRSumVariant=Passthrough  SumFdbkVariant=Disabled  SumVariant=Sum_PID
  Roll : Outport  VectorParamsAs1DForOutWhenUnconnected=off
  Pitch : Outport  Port=2  VectorParamsAs1DForOutWhenUnconnected=off
  Yaw : Outport  Port=3  VectorParamsAs1DForOutWhenUnconnected=off
  error : Outport  Port=4
  pid_p_comand : Outport  Port=5
  wires:
  r/1 -> "          "/1
  Mux22/1 -> Demux16/1
  yaw_rate/1 -> Yaw/1
  "          "/1 -> Sum17/1
  roll_rate/1 -> Roll/1
  Sum19/1 -> pitch_attitude/1
  pitch_attitude/1 -> Mux22/2
  roll_attitude/1 -> Mux22/1
  Demux16/1 -> pid_p_comand/1, Sum21/2
  yaw/1 -> Sum17/2
  roll_pitch/1 -> Demux12/1
  Demux16/2 -> Sum22/2
  Demux12/1 -> Sum18/2
  Demux12/2 -> Sum19/2
  phi/1 -> Sum18/1
  theta/1 -> Sum19/1
  Sum18/1 -> error/1, roll_attitude/1
  pitch_rate/1 -> Pitch/1
  Sum22/1 -> pitch_rate/1
  Sum17/1 -> yaw_rate/1
  p/1 -> Sum21/1
  q/1 -> Sum22/1
  Sum21/1 -> roll_rate/1

== system quadFly/Control System1/InputConditioning ==
  roll : Inport
  pitch : Inport  Port=2
  thrust : Inport  Port=3
  yaw : Inport  Port=4
  Demux : Demux  Outputs=2
  Fcn2 : Fcn  Expr=(u - 1500) / 800
  Fcn5 : Fcn  Expr=(u - 1500) / 800
  Fcn6 : Fcn  Expr=(u - 1100) / 800
  Fcn7 : Fcn  Expr=(u - 1500) / 800
  Gain : Gain  Gain=MAX_CONTROL_ANGLE_RATE_Y
  Gain2 : Gain  Gain=3.1415  OutDataTypeStr=Inherit: Inherit via back propagation
  MATLAB Function : MATLAB Function  TreatAsAtomicUnit=on
  MATLAB Function1 : MATLAB Function  TreatAsAtomicUnit=on
  MATLAB Function2 : MATLAB Function  TreatAsAtomicUnit=on
  MATLAB Function3 : MATLAB Function  TreatAsAtomicUnit=on
  Mux21 : Mux  Inputs=2
  Saturation10 : Saturate  UpperLimit=1  LowerLimit=0
  Saturation7 : Saturate  UpperLimit=1  LowerLimit=-1
  Saturation8 : Saturate  UpperLimit=1  LowerLimit=-1
  Saturation9 : Saturate  UpperLimit=1/2  LowerLimit=-1/2
  Roll_Pitch : Outport  VectorParamsAs1DForOutWhenUnconnected=off
  Yaw : Outport  Port=2  VectorParamsAs1DForOutWhenUnconnected=off
  Thrust : Outport  Port=3  VectorParamsAs1DForOutWhenUnconnected=off
  Out Bus Element : Outport  Port=4  PortName=OutBus  Element=roll_comand
  Out Bus Element1 : Outport  Port=4  PortName=OutBus  Element=signal2
  wires:
  Saturation10/1 -> Thrust/1
  Saturation7/1 -> Gain/1
  Gain2/1 -> Demux/1, Roll_Pitch/1
  Mux21/1 -> Gain2/1
  Saturation8/1 -> Mux21/2
  Fcn6/1 -> Saturation10/1
  Fcn2/1 -> Saturation9/1
  Fcn5/1 -> Saturation8/1
  Saturation9/1 -> Mux21/1
  Fcn7/1 -> Saturation7/1
  pitch/1 -> MATLAB Function2/1(u)
  MATLAB Function1/1(y) -> Fcn7/1
  thrust/1 -> MATLAB Function3/1(u)
  roll/1 -> MATLAB Function/1(u)
  MATLAB Function2/1(y) -> Fcn5/1
  MATLAB Function/1(y) -> Fcn2/1
  yaw/1 -> MATLAB Function1/1(u)
  MATLAB Function3/1(y) -> Fcn6/1
  Gain/1 -> Yaw/1
  Demux/1 -> Out Bus Element/1
  Demux/2 -> Out Bus Element1/1

== system quadFly/Control System1/LED  ==
  In1 : Inport
  Compare To Constant3 : simulink/Logic and Bit Operations/Compare To Constant  relop=>=  const=uint16(1500)  OutDataTypeStr=boolean
  Out1 : Outport  VectorParamsAs1DForOutWhenUnconnected=off
  wires:
  Compare To Constant3/1 -> Out1/1
  In1/1 -> Compare To Constant3/1

== system quadFly/Quadcopter Dynamics/6DOF ==
  Force and Moment Model Bus : Inport
  Fail Model Bus : Inport  Port=2
  Bus Creator : BusCreator  Inputs=7
  Bus Selector : BusSelector  OutputSignals=dM,m,J
  Bus Selector1 : BusSelector  OutputSignals=Fb,Mb
  Constant_dI/dt : Constant  Value=zeros(3,3)
  Custom Variable Mass 6DOF (Quaternion) : shared6dof/6DOF (Euler Angles)  units=Metric (MKS)  mtype=Custom Variable  rep=Quaternion  xme_0=ModelInit_PosE  Vm_0=ModelInit_VelB  eul_0=ModelInit_AngEuler  pm_0=ModelInit_RateB  mass_0=1.0  mass_e=0.5  mass_f=2.0  inertia=eye(3)  inertia_e=eye(3)  inertia_f=2*eye(3)  k_quat=1.0  vre_flag=off  abi_flag=off  aMode=aMode  xme_statename=''  Vm_statename=''  eul_statename=''  quat_statename=''  pm_statename=''  mass_statename=''
      settings: SourceProductBaseCode=AE
  Sum : Sum  Inputs=++|
  Terminator : Terminator
  6DOF Bus : Outport  VectorParamsAs1DForOutWhenUnconnected=off
  wires:
  Bus Selector1/1 -> Custom Variable Mass 6DOF (Quaternion)/1  "<Fb>"
  Bus Selector/2 -> Custom Variable Mass 6DOF (Quaternion)/3  "<m>"
  Custom Variable Mass 6DOF (Quaternion)/8 -> Terminator/1
  Sum/1 -> Custom Variable Mass 6DOF (Quaternion)/2
  Constant_dI/dt/1 -> Custom Variable Mass 6DOF (Quaternion)/4
  Custom Variable Mass 6DOF (Quaternion)/5 -> Bus Creator/5  "Vb"
  Custom Variable Mass 6DOF (Quaternion)/6 -> Bus Creator/6  "wb"
  Custom Variable Mass 6DOF (Quaternion)/1 -> Bus Creator/1  "Ve"
  Custom Variable Mass 6DOF (Quaternion)/4 -> Bus Creator/4  "DCM"
  Custom Variable Mass 6DOF (Quaternion)/2 -> Bus Creator/2  "Xe"
  Custom Variable Mass 6DOF (Quaternion)/3 -> Bus Creator/3  "Eular(rad)"
  Custom Variable Mass 6DOF (Quaternion)/7 -> Bus Creator/7  "dwb/dt"
  Bus Selector/3 -> Custom Variable Mass 6DOF (Quaternion)/5  "<J>"
  Bus Selector/1 -> Sum/2  "<dM>"
  Bus Selector1/2 -> Sum/1  "<Mb>"
  Fail Model Bus/1 -> Bus Selector/1
  Force and Moment Model Bus/1 -> Bus Selector1/1
  Bus Creator/1 -> 6DOF Bus/1

== system quadFly/Quadcopter Dynamics/Battery Model ==
  PWMin : Inport
  Battery Model_sfcn : S-Function  FunctionName=Battery_sf  SFunctionModules=""  SFunctionDeploymentMode=off  EnableBusSupport=off  mask{rtw_sf_name=Battery_sf, showVar=off}
      mask prompts: rtw_sf_name "Simulink:masks:GenSFuncName_MP"; showVar "Simulink:masks:GenSFuncShowModuleList_MP"
      mask help: Simulink:masks:GenSFuncDesc_MD
      mask init:
      | displist = '';
      | if ~strcmp(get_param(gcb, 'FunctionName'), rtw_sf_name);
      |   set_param(gcb, 'FunctionName', rtw_sf_name);
      | end
      | % Check if we are generating code
      | rtw_mode = false;
      | if strcmpi(get_param(bdroot(gcb),'SimulationStatus'),'Initializing')
      | 	rtw_mode = strcmpi(get_param(bdroot(gcb),'BuildingRTWCode'),'on') && ...
      | 		~strcmpi(get_param(bdroot(gcb),'TargetStyle'),'SimulationTarget');
      | end
      | if showVar || rtw_mode
      | 	if exist('rtwsfunc') == 2 | exist('rtwsfunc') == 6
      | 		tmplist = rtwsfunc(rtw_sf_name,gcb);
      | 		tmplist = DAStudio.message('Simulink:masks:GenSFuncListOfModules_IC', tmplist);
      | 	elseif showVar
      | 		tmplist1 = DAStudio.message('Simulink:masks:GenSFuncListOfModules_IC', '');
      |         tmplist2 = DAStudio.message('Simulink:masks:GenSFuncNotLicensed_IC');
      |         tmplist = [tmplist1 tmplist2];
      |  	end
      | end
      | if showVar
      |   displist = tmplist;
      | end
      settings: CopyFcn=|
      | if ~strcmp(get_param(gcb,'Linkstatus'),'none') && ...
      | ~strcmp(get_param(gcb,'Linkstatus'),'implicit')
      |   set_param(gcb,'LinkStatus','none');
      | end
      mask Help: eval('feval(''rtwprivate'',''rtwhelpview'',''rtw_sfcn_block'')');
      mask Display:
      | port_label('input',1,'PWMin');
      | port_label('output',1,'PWMOut');
      | port_label('output',2,'cellVol');
      | port_label('output',3,'remCapa');
  __InputSSForSFun__ : Subsystem
  __OutputSSForSFun__ : Subsystem
  Battery Model Bus : Outport  VectorParamsAs1DForOutWhenUnconnected=off
  wires:
  PWMin/1 -> __InputSSForSFun__/1(PWMin)
  __InputSSForSFun__/1(__UniqueOutportName__1__) -> Battery Model_sfcn/1
  Battery Model_sfcn/1 -> __OutputSSForSFun__/1(__UniqueInportName__1__)
  Battery Model_sfcn/2 -> __OutputSSForSFun__/2(__UniqueInportName__2__)
  Battery Model_sfcn/3 -> __OutputSSForSFun__/3(__UniqueInportName__3__)
  __OutputSSForSFun__/1(Battery Model Bus) -> Battery Model Bus/1

== system quadFly/Quadcopter Dynamics/Environment Model ==
  6DOF Bus : Inport
  Environment Model_sfcn : S-Function  FunctionName=Environment_sf  Parameters=sfcnParam1, sfcnParam2, sfcnParam3  SFunctionModules=""  SFunctionDeploymentMode=off  EnableBusSupport=off  SFcnStateName=DWORK0,DWORK1,DWORK2,DWORK3,DWORK4,DWORK5,DWORK6,DWORK7,DWORK8,DWORK9,DWORK10,DWORK11,DWORK12,DWORK13,DWORK14,DWORK15  mask{rtw_sf_name=Environment_sf, showVar=off, sfcnParam1=sfcnParam1, sfcnParam2=sfcnParam2, sfcnParam3=sfcnParam3}
      mask prompts: rtw_sf_name "Simulink:masks:GenSFuncName_MP"; showVar "Simulink:masks:GenSFuncShowModuleList_MP"; sfcnParam1 "ModelParam_GPSLatLong:"; sfcnParam2 "ModelParam_GlobalNoiseGainSwitch:"; sfcnParam3 "ModelParam_envAltitude:"
      mask help: Simulink:masks:GenSFuncDesc_MD
      mask init: same as quadFly/Quadcopter Dynamics/Battery Model/Battery Model_sfcn
      settings: SFcnIsStateOwnerBlock=on
      settings: CopyFcn=|
      | if ~strcmp(get_param(gcb,'Linkstatus'),'none') && ...
      | ~strcmp(get_param(gcb,'Linkstatus'),'implicit')
      |   set_param(gcb,'LinkStatus','none');
      | end
      mask Help: eval('feval(''rtwprivate'',''rtwhelpview'',''rtw_sfcn_block'')');
      mask Display:
      | port_label('input',1,'Ve');
      | port_label('input',2,'Xe');
      | port_label('input',3,'Eular(rad)');
      | port_label('input',4,'DCM');
      | port_label('input',5,'Vb');
      | port_label('input',6,'wb');
      | port_label('input',7,'dwb/dt');
      | port_label('output',1,'PosGPS');
      | port_label('output',2,'gravity');
      | port_label('output',3,'TempC');
      | port_label('output',4,'AirPressure');
      | port_label('output',5,'Rho');
      | port_label('output',6,'Windb');
      | port_label('output',7,'Wind');
  __InputSSForSFun__ : Subsystem
  __OutputSSForSFun__ : Subsystem
  Environment Model Bus : Outport  VectorParamsAs1DForOutWhenUnconnected=off
  wires:
  6DOF Bus/1 -> __InputSSForSFun__/1(6DOF Bus)
  __InputSSForSFun__/1(__UniqueOutportName__1__) -> Environment Model_sfcn/1
  __InputSSForSFun__/2(__UniqueOutportName__2__) -> Environment Model_sfcn/2
  __InputSSForSFun__/3(__UniqueOutportName__3__) -> Environment Model_sfcn/3
  __InputSSForSFun__/4(__UniqueOutportName__4__) -> Environment Model_sfcn/4
  __InputSSForSFun__/5(__UniqueOutportName__5__) -> Environment Model_sfcn/5
  __InputSSForSFun__/6(__UniqueOutportName__6__) -> Environment Model_sfcn/6
  __InputSSForSFun__/7(__UniqueOutportName__7__) -> Environment Model_sfcn/7
  Environment Model_sfcn/1 -> __OutputSSForSFun__/1(__UniqueInportName__1__)
  Environment Model_sfcn/2 -> __OutputSSForSFun__/2(__UniqueInportName__2__)
  Environment Model_sfcn/3 -> __OutputSSForSFun__/3(__UniqueInportName__3__)
  Environment Model_sfcn/4 -> __OutputSSForSFun__/4(__UniqueInportName__4__)
  Environment Model_sfcn/5 -> __OutputSSForSFun__/5(__UniqueInportName__5__)
  Environment Model_sfcn/6 -> __OutputSSForSFun__/6(__UniqueInportName__6__)
  Environment Model_sfcn/7 -> __OutputSSForSFun__/7(__UniqueInportName__7__)
  __OutputSSForSFun__/1(Environment Model Bus) -> Environment Model Bus/1
